simulink model "EcoSIM3_P2_C2_WIP"  (R2014b)
settings: Solver=ode1  SolverMode=SingleTasking  StartTime=0.0  StopTime=4  FixedStep=0.01  RelTol=1e-3
PostLoadFcn:
  | %, if any(exist('dsrtsu_mdlpostloadfcn', 'file') == [2, 3, 6]), try dsrtsu_mdlpostloadfcn('Execute', bdroot); catch fprintf('Error in PostLoadFcn (dsrtsu_mdlpostloadfcn) for model "%s":\n %s\n', bdroot, lasterr); end, end,
InitFcn:
  | tic
  | %Startup_EcoSIM
undefined symbols (not defined in the file or in its folder): canChannel, Controls, DriveCycles, Driver, EM_EFF_MAP, EM_PwrLoss_MAP, EngPwr, EngSpd, EngTrq, Glbl, Overwritten_Mode, Plants, Power, sigbuilder_block, Torque, Trialmap, Veh_Dynamics
libraries: simulink x135, canmsglib x113, fl_lib x104, canlib x89, nesl_utility x56, sdl_lib x29, dspsigops x6, dspswit3 x5, dspstat3 x2, commnoisgen2 x1, dspfdesign x1
(part 6 of 21)

== system EcoSIM3_P2_C2_WIP/Powertrain/Clutch_Transmission1/Mastershift Softecu/Algorithm ==
  note: Cignals getting transmitted to Actuators are bussed together here
  note: Sensor signals getting transmitted over CAN are selected here
  note: Signals like T& E are used to calculate whatever is required by Soft ECU
  Inputs : Inport
  Add4 : Sum
  Bus Creator : BusCreator  Inputs=2
  Bus Selector : BusSelector  OutputSignals=Clutch_Sw,Sensor_Out.Trans_Sensor_Out.Actual_Gear,Upshift_Sw,Downshift_Sw
  Chart : Stateflow chart  TreatAsAtomicUnit=on
  Display : Display
  Display1 : Display
  Downshift Counter : dspswit3/Counter  Direction=Up  CountEvent=Rising edge  CounterSize=User defined  MaxCount=255  InitialCount=0  Output=Count  HitValue=32  ResetInput=on  SamplesPerFrame=1  Ts=1  CntDtype=double  HitDtype=Logical
  Gain : Gain  Gain=-1
  Memory : Memory
  Memory1 : Memory
  Upshift Counter : dspswit3/Counter  Direction=Up  CountEvent=Rising edge  CounterSize=User defined  MaxCount=255  InitialCount=0  Output=Count  HitValue=32  ResetInput=on  SamplesPerFrame=1  Ts=1  CntDtype=double  HitDtype=Logical
  Outputs : Outport
  wires:
  Chart/1(Gear_Cmd) -> Bus Creator/1, Display/1
  Memory1/1 -> Upshift Counter/2, Downshift Counter/2
  Bus Creator/1 -> Outputs/1
  Memory/1 -> Chart/2(Actual_Gear)
  Chart/3(reset) -> Memory1/1  "reset"
  Add4/1 -> Display1/1, Chart/3(Count)
  Bus Selector/4 -> Downshift Counter/1  "<Downshift_Sw>"
  Bus Selector/3 -> Upshift Counter/1  "<Upshift_Sw>"
  Gain/1 -> Add4/2
  Downshift Counter/1 -> Gain/1
  Upshift Counter/1 -> Add4/1
  Chart/2(TCM_Gear) -> Bus Creator/2  "TCM_Gear"
  Bus Selector/1 -> Chart/1(Clutch_Sw)  "<Clutch_Sw>"
  Bus Selector/2 -> Memory/1  "<Actual_Gear>"
  Inputs/1 -> Bus Selector/1

== system EcoSIM3_P2_C2_WIP/Powertrain/Clutch_Transmission1/Mastershift Softecu/Inputs ==
  note: Combine all the Signals that go to the
      | Soft ECU Algorithm:
      | -Calculated Signals from Sensors and CAN
      | -Signalfrom sensors pass through because they
      | need to be sent out over the CAN by the ECU
  note: Select the Sensor signals
  note: Select the CAN signals
  note: Do the input conditioning (if any) required by the
      | Algorith
  Sensors : Inport
  From GCM : Inport  Port=2
  Clutch_CAN_Out : Inport  Port=3
  Bus Creator : BusCreator
  Bus Selector : BusSelector  OutputSignals=Upshift_Sw,Downshift_Sw
  Bus Selector1 : BusSelector  OutputSignals=Clutch_Sw
  To_Algorithm : Outport
  wires:
  Bus Selector/2 -> Bus Creator/3  "<Downshift_Sw>"
  Bus Selector/1 -> Bus Creator/2  "<Upshift_Sw>"
  Bus Selector1/1 -> Bus Creator/4  "<Clutch_Sw>"
  Clutch_CAN_Out/1 -> Bus Selector1/1
  Bus Creator/1 -> To_Algorithm/1  "Component_to_Alg"
  Sensors/1 -> Bus Creator/1
  From GCM/1 -> Bus Selector/1

== system EcoSIM3_P2_C2_WIP/Powertrain/Clutch_Transmission1/Mastershift Softecu/Outputs ==
  note: Combine all the Signals that go to the
      | Soft ECU Algorithm:
      | -Calculated Signals from Sensors and CAN
      | -Signalfrom sensors pass through because they
      | need to be sent out over the CAN by the ECU
  From Algorithm : Inport
  Bus Creator : BusCreator  Inputs=1
  Bus Selector : BusSelector  OutputSignals=Gear_Cmd,TCM_Gear
  Actuator Commands : Outport
  To GCM : Outport  Port=2
  wires:
  Bus Creator/1 -> Actuator Commands/1  "Trans_Actuator_Commands"
  Bus Selector/2 -> To GCM/1  "<TCM_Gear>"
  Bus Selector/1 -> Bus Creator/1  "<Gear_Cmd>"
  From Algorithm/1 -> Bus Selector/1

== system EcoSIM3_P2_C2_WIP/Powertrain/Clutch_Transmission1/Trans_Plant/Actuators ==
  note: Actuator Model or a Signal Pass-through, Remove the bus if you are passing through all the signals
  ActuatorInputs : Inport
  Actuator Outputs : Outport
  wires:
  ActuatorInputs/1 -> Actuator Outputs/1

== system EcoSIM3_P2_C2_WIP/Powertrain/Clutch_Transmission1/Trans_Plant/Plant ==
  note: Component Level Performance Maps
  note: Try to detect actual gears from simscape model. Using reverse lookup from rate limiter starts giving value from Gear 5, because it has the lowest ratio
  From_Actuators : Inport
  Bus Selector : BusSelector  OutputSignals=Clutch_Trans_SoftECU_Receive.Clutch_Trans_CAN.Trans_Receive.Gear_Request
  Input Shaft Inertia : fl_lib/Mechanical/Rotational Elements/Inertia  inertia=0.01 kg*m^2  w_specify=off  w_priority=High  w=580*2*pi/60 rad/s  t_specify=off  t_priority=High  t=0 N*m
  Output Shaft Inertia1 : fl_lib/Mechanical/Rotational Elements/Inertia  inertia=.01 kg*m^2  w_specify=off  w_priority=High  w=580*2*pi/60 rad/s  t_specify=off  t_priority=High  t=0 N*m
  Rate Limiter : RateLimiter  RisingSlewLimit=2  FallingSlewLimit=-2  SampleTimeMode=inherited  InitialCondition=2.95
  ReverseLookup : Lookup  InputValues=[0 0.6300 1 1.3400 1.9400 2.9500]  Table=[0 5 4 3 2 1]  LookUpMeth=Use Input Nearest
  Simulink-PS Converter : nesl_utility/Simulink-PS Converter  PhysicalDomain=network_engine_domain  SubClassName=ps_input  LeftPortType=input  RightPortType=output  PseudoPeriodic=off  Frequencies=[]  NoiseDistribution=none  NoiseParameters=[]  Unit=1  AffineConversion=off  InputFiltering=off  SimscapeFilterOrder=1  InputFilterTimeConstant=0.001  UdotUserProvided=1
  Trans GR : Lookup  InputValues=Plants.Trans.Mdl.Plant.Gear_cmd  Table=Plants.Trans.Mdl.Plant.GR  LookUpMeth=Use Input Nearest
  Variable Ratio Transmission : sdl_lib/Couplings & Drives/Variable Ratio Transmission  rotation_direction=1  kp=3e+5 N*m/rad  kv=0.05 N*m/(rad/s)  initial_torque=0 N*m  losses_model=1  efficiency=0.8  mu_visc=[ 0 0 ] N*m/(rad/s)  w_thr=0.01 rad/s
  Trans Input Shaft : PMIOPort  Port=1  Side=Left
  To Sensors : PMIOPort  Port=2  Side=Right
  Actual_Gear : Outport
  wires:
  Rate Limiter/1 -> Simulink-PS Converter/1, ReverseLookup/1
  Trans GR/1 -> Rate Limiter/1
  ReverseLookup/1 -> Actual_Gear/1
  From_Actuators/1 -> Bus Selector/1
  Bus Selector/1 -> Trans GR/1  "<Gear_Request>"
  connections:
  Simulink-PS Converter/RConn1 -- Variable Ratio Transmission/LConn1
  To Sensors/RConn1 -- Output Shaft Inertia1/LConn1 -- Variable Ratio Transmission/RConn1
  Variable Ratio Transmission/LConn2 -- Input Shaft Inertia/LConn1 -- Trans Input Shaft/RConn1

== system EcoSIM3_P2_C2_WIP/Powertrain/Clutch_Transmission1/Trans_Plant/Sensors ==
  note: Sensor Model: Place where we add Corrupter
  Actual_Gear : Inport
  Bus Creator : BusCreator  Inputs=3
  Ideal Rotational Motion Sensor : fl_lib/Mechanical/Mechanical Sensors/Ideal Rotational Motion Sensor  offset=0 rad
  Ideal Torque Sensor : fl_lib/Mechanical/Mechanical Sensors/Ideal Torque Sensor
  Mechanical Rotational Reference1 : fl_lib/Mechanical/Rotational Elements/Mechanical Rotational Reference
  PS-Simulink Converter : nesl_utility/PS-Simulink Converter  PhysicalDomain=network_engine_domain  SubClassName=ps_output  LeftPortType=input  RightPortType=output  PseudoPeriodic=off  Frequencies=[]  Unit=1  AffineConversion=off
  PS-Simulink Converter1 : nesl_utility/PS-Simulink Converter  PhysicalDomain=network_engine_domain  SubClassName=ps_output  LeftPortType=input  RightPortType=output  PseudoPeriodic=off  Frequencies=[]  Unit=N*m  AffineConversion=off
  Trans Output Shaft : PMIOPort  Port=1  Side=Left
  To_MC : PMIOPort  Tag=PMCPort  Port=2  Side=Right
  Sensor Out : Outport
  ActGear : Outport  Port=2
  wires:
  Actual_Gear/1 -> Bus Creator/1, ActGear/1  "Actual_Gear"
  PS-Simulink Converter/1 -> Bus Creator/2  "Trans_Speed_rad_per_s"
  PS-Simulink Converter1/1 -> Bus Creator/3  "Trans_Torque_Out_Nm"
  Bus Creator/1 -> Sensor Out/1  "Trans_Sensor"
  connections:
  Ideal Torque Sensor/LConn1 -- Ideal Rotational Motion Sensor/LConn1 -- Trans Output Shaft/RConn1
  Ideal Rotational Motion Sensor/RConn1 -- Mechanical Rotational Reference1/LConn1
  PS-Simulink Converter1/LConn1 -- Ideal Torque Sensor/RConn2
  PS-Simulink Converter/LConn1 -- Ideal Rotational Motion Sensor/RConn2
  To_MC/RConn1 -- Ideal Torque Sensor/RConn1

== system EcoSIM3_P2_C2_WIP/Powertrain/Clutch_Transmission2/CP1 SoftEcu/Algorithm ==
  note: Cignals getting transmitted to Actuators are bussed together here
  note: Sensor signals getting transmitted over CAN are bussed together here
  note: Sensor signals getting transmitted over CAN are selected here
  note: Signals like T& E are used to calculate whatever is required by Soft ECU
  note: SpA position 0 to 6327
      | 0 = Fully Engaged
      | 6327 = Fully Disengaged
  Inputs : Inport
  Add : Sum  Inputs=-+
  Bus Creator2 : BusCreator
  Bus Selector : BusSelector  OutputSignals=CP1_SoftECU_Receive.CP1_CAN.MSG_HYB_15.MY15_CCU_posDes,Sensor_Out.Clutch_Sensor_Out.Clutch_Pressure
  Chart : Stateflow chart  TreatAsAtomicUnit=on
  Constant : Constant
  Gain : Gain  Gain=1/6327
  Gain1 : Gain  Gain=1/(4400000*0.4)
  Gain2 : Gain  Gain=6327
  Ground : Ground
  Scope : Scope
      settings: SaveName=ScopeData51
  Scope1 : Scope
      settings: SaveName=ScopeData52
  Outputs : Outport
  wires:
  Inputs/1 -> Bus Selector/1
  Bus Selector/1 -> Scope1/1, Chart/1(Position_Request)  "<MY15_CCU_posDes>"
  Chart/2(Mode) -> Bus Creator2/2  "CY01_stMode"
  Chart/1(Position_Command) -> Gain/1
  Gain/1 -> Bus Creator2/1  "SpA_Position_Command"
  Gain1/1 -> Add/1
  Bus Selector/2 -> Gain1/1  "<Clutch_Pressure>"
  Gain2/1 -> Scope/1, Bus Creator2/3  "CY01_posCurr"
  Ground/1 -> Bus Creator2/4  "Dummy_Electrical1"
  Bus Creator2/1 -> Outputs/1  "CP1_SoftECU_Out"
  Add/1 -> Gain2/1
  Constant/1 -> Add/2

== system EcoSIM3_P2_C2_WIP/Powertrain/Clutch_Transmission2/CP1 SoftEcu/Inputs ==
  note: Combine all the Signals that go to the
      | Soft ECU Algorithm:
      | -Calculated Signals from Sensors and CAN
      | -Signalfrom sensors pass through because they
      | need to be sent out over the CAN by the ECU
  note: Select the Sensor signals
  note: Select the CAN signals
  note: Do the input conditioning (if any) required by the
      | Algorith
  Sensors : Inport
  CAN : Inport  Port=2
  Bus Creator : BusCreator  Inputs=2
  Bus Selector : BusSelector  OutputSignals=CP1_SoftECU_Receive
  To_Algorithm : Outport
  wires:
  Bus Creator/1 -> To_Algorithm/1  "Component_to_Alg"
  Sensors/1 -> Bus Creator/1  "Sensor_Out"
  CAN/1 -> Bus Selector/1
  Bus Selector/1 -> Bus Creator/2  "<CP1_SoftECU_Receive>"

== system EcoSIM3_P2_C2_WIP/Powertrain/Clutch_Transmission2/CP1 SoftEcu/Outputs ==
  From Algorithm : Inport
  Bus Creator : BusCreator  Inputs=1
  Bus Creator1 : BusCreator  Inputs=3
  Bus Selector1 : BusSelector  OutputSignals=SpA_Position_Command,CY01_stMode,CY01_posCurr,Dummy_Electrical1
  Actuator Cmd : Outport
  CAN : Outport  Port=2
  wires:
  From Algorithm/1 -> Bus Selector1/1  "Sensor_Out"
  Bus Selector1/1 -> Bus Creator/1  "<SpA_Position_Command>"
  Bus Creator/1 -> Actuator Cmd/1  "Component_Actuator_Commands"
  Bus Selector1/3 -> Bus Creator1/2  "<CY01_posCurr>"
  Bus Selector1/4 -> Bus Creator1/3  "<Dummy_Electrical1>"
  Bus Selector1/2 -> Bus Creator1/1  "<CY01_stMode>"
  Bus Creator1/1 -> CAN/1  "CP1_Out"

== system EcoSIM3_P2_C2_WIP/Powertrain/Clutch_Transmission2/Clutch_Plant/Custom Clutch ==
  -1 : fl_lib/Physical Signals/Functions/PS Gain  gain=-1
  Dynamic friction coefficient lookup table : fl_lib/Physical Signals/Lookup Tables/PS Lookup Table (1D)  x_t=[ 0 0.1 0.2 0.3 0.4 0.5 1 2 5 10 100 1000 ]  y_t=[ 0.29 0.28 0.26 0.22 0.21 0.2 0.2 0.19 0.19 0.19 0.19 0.19 ]  interp_method=1  extrap_method=1
  Effective radius : fl_lib/Physical Signals/Functions/PS Gain  gain=0.3
  Fundamental Friction Clutch : sdl_lib/Clutches/Fundamental Components/Fundamental Friction Clutch  unidirectional=0  w_tol=0.001 rad/s  initial_state_locked=0
  PS Abs : fl_lib/Physical Signals/Nonlinear Operators/PS Abs
  PS Product1 : fl_lib/Physical Signals/Functions/PS Product
  PS-Simulink Converter1 : nesl_utility/PS-Simulink Converter  PhysicalDomain=network_engine_domain  SubClassName=ps_output  LeftPortType=input  RightPortType=output  PseudoPeriodic=off  Frequencies=[]  Unit=rad/s  AffineConversion=off
  Peak force : fl_lib/Physical Signals/Functions/PS Gain  gain=10
  Slip(rad/s) : Scope
      settings: YMin=-4  YMax=1
  Static/dynamic friction ratio : fl_lib/Physical Signals/Functions/PS Gain  gain=1.1
  "[0, inf]" : fl_lib/Physical Signals/Nonlinear Operators/PS Saturation  upper_limit=inf  lower_limit=0
  P : PMIOPort  Port=1  Side=Left
  Mode : PMIOPort  Port=2  Side=Right
  F : PMIOPort  Port=3  Side=Right
  B : PMIOPort  Port=4  Side=Left
  wires:
  PS-Simulink Converter1/1 -> Slip(rad/s)/1
  connections:
  Peak force/RConn1 -- PS Product1/LConn1
  PS Product1/RConn1 -- Effective radius/LConn1
  "[0, inf]"/RConn1 -- Peak force/LConn1
  Fundamental Friction Clutch/RConn3 -- F/RConn1
  Fundamental Friction Clutch/RConn2 -- Mode/RConn1
  PS-Simulink Converter1/LConn1 -- Fundamental Friction Clutch/RConn1 -- PS Abs/LConn1
  B/RConn1 -- Fundamental Friction Clutch/LConn4
  P/RConn1 -- "[0, inf]"/LConn1
  Fundamental Friction Clutch/LConn2 -- -1/LConn1 -- Static/dynamic friction ratio/RConn1
  Effective radius/RConn1 -- Fundamental Friction Clutch/LConn1 -- Static/dynamic friction ratio/LConn1
  Dynamic friction coefficient lookup table/RConn1 -- PS Product1/LConn2
  -1/RConn1 -- Fundamental Friction Clutch/LConn3
  PS Abs/RConn1 -- Dynamic friction coefficient lookup table/LConn1

== system EcoSIM3_P2_C2_WIP/Powertrain/Clutch_Transmission2/Clutch_Plant/Sensors ==
  Clutch_Pressure : Inport
  Bus Creator : BusCreator  Inputs=1
  Ideal Rotational Motion Sensor : fl_lib/Mechanical/Mechanical Sensors/Ideal Rotational Motion Sensor  offset=0 rad
  Ideal Torque Sensor : fl_lib/Mechanical/Mechanical Sensors/Ideal Torque Sensor
  Mechanical Rotational Reference1 : fl_lib/Mechanical/Rotational Elements/Mechanical Rotational Reference
  PS-Simulink Converter : nesl_utility/PS-Simulink Converter  PhysicalDomain=network_engine_domain  SubClassName=ps_output  LeftPortType=input  RightPortType=output  PseudoPeriodic=off  Frequencies=[]  Unit=rad/s  AffineConversion=off
  PS-Simulink Converter1 : nesl_utility/PS-Simulink Converter  PhysicalDomain=network_engine_domain  SubClassName=ps_output  LeftPortType=input  RightPortType=output  PseudoPeriodic=off  Frequencies=[]  Unit=N*m  AffineConversion=off
  Terminator : Terminator
  Terminator1 : Terminator
  Shaft : PMIOPort  Port=1  Side=Left
  To_Trans : PMIOPort  Tag=PMCPort  Port=2  Side=Right
  Clutch_Status : Outport
  wires:
  PS-Simulink Converter/1 -> Terminator/1  "Clutch_Speed_rad_per_s"
  PS-Simulink Converter1/1 -> Terminator1/1  "Clutch_Torque_Out_Nm"
  Clutch_Pressure/1 -> Bus Creator/1  "Clutch_Pressure"
  Bus Creator/1 -> Clutch_Status/1  "Clutch_Sensor_Out"
  connections:
  Ideal Torque Sensor/LConn1 -- Shaft/RConn1 -- Ideal Rotational Motion Sensor/LConn1
  Ideal Rotational Motion Sensor/RConn1 -- Mechanical Rotational Reference1/LConn1
  PS-Simulink Converter/LConn1 -- Ideal Rotational Motion Sensor/RConn2
  PS-Simulink Converter1/LConn1 -- Ideal Torque Sensor/RConn2
  To_Trans/RConn1 -- Ideal Torque Sensor/RConn1

== system EcoSIM3_P2_C2_WIP/Powertrain/Clutch_Transmission2/Mastershift Softecu/Algorithm ==
  note: Signals like T& E are used to calculate whatever is required by Soft ECU
  note: Sensor signals getting transmitted over CAN are selected here
  note: Cignals getting transmitted to Actuators are bussed together here
  Inputs : Inport
  Add4 : Sum
  Bus Creator : BusCreator  Inputs=3
  Bus Selector : BusSelector  OutputSignals=Mastershift_SoftECU_Receive.Mastershift_Electrical.Clutch_Sw,Sensor_Out.Trans_Sensor_Out.Actual_Gear,Mastershift_SoftECU_Receive.Mastershift_Electrical.Upshift_Sw,Mastershift_SoftECU_Receive.Mastershift_Electrical.Downshift_Sw
  Chart : Stateflow chart  TreatAsAtomicUnit=on
  Display : Display
  Display1 : Display
  Downshift Counter : dspswit3/Counter  Direction=Up  CountEvent=Rising edge  CounterSize=User defined  MaxCount=255  InitialCount=0  Output=Count  HitValue=32  ResetInput=on  SamplesPerFrame=1  Ts=1  CntDtype=double  HitDtype=Logical
  Gain : Gain  Gain=-1
  Ground : Ground
  Memory : Memory
  Memory1 : Memory
  Scope : Scope
      settings: SaveName=ScopeData30
  Scope1 : Scope
      settings: SaveName=ScopeData31
  Scope2 : Scope
      settings: SaveName=ScopeData48
  Upshift Counter : dspswit3/Counter  Direction=Up  CountEvent=Rising edge  CounterSize=User defined  MaxCount=255  InitialCount=0  Output=Count  HitValue=32  ResetInput=on  SamplesPerFrame=1  Ts=1  CntDtype=double  HitDtype=Logical
  Outputs : Outport
  wires:
  Inputs/1 -> Bus Selector/1
  Bus Selector/2 -> Memory/1  "<Actual_Gear>"
  Bus Selector/1 -> Chart/1(Clutch_Sw)  "<Clutch_Sw>"
  Chart/2(TCM_Gear) -> Bus Creator/2  "Mastershift_Gear"
  Upshift Counter/1 -> Add4/1
  Downshift Counter/1 -> Gain/1
  Gain/1 -> Add4/2
  Bus Selector/3 -> Scope/1, Upshift Counter/1  "<Upshift_Sw>"
  Bus Selector/4 -> Downshift Counter/1  "<Downshift_Sw>"
  Add4/1 -> Scope1/1, Chart/3(Count), Display1/1
  Chart/3(reset) -> Memory1/1  "reset"
  Memory/1 -> Chart/2(Actual_Gear)
  Bus Creator/1 -> Outputs/1  "Mastershift_SoftECU_Out"
  Memory1/1 -> Downshift Counter/2, Upshift Counter/2
  Chart/1(Gear_Cmd) -> Scope2/1, Bus Creator/1, Display/1
  Ground/1 -> Bus Creator/3  "Dummy_Electrical1"

== system EcoSIM3_P2_C2_WIP/Powertrain/Clutch_Transmission2/Mastershift Softecu/Inputs ==
  note: Do the input conditioning (if any) required by the
      | Algorith
  note: Select the CAN signals
  note: Select the Sensor signals
  note: Combine all the Signals that go to the
      | Soft ECU Algorithm:
      | -Calculated Signals from Sensors and CAN
      | -Signalfrom sensors pass through because they
      | need to be sent out over the CAN by the ECU
  Sensors : Inport
  CAN : Inport  Port=2
  Bus Creator : BusCreator  Inputs=2
  Bus Selector : BusSelector  OutputSignals=Mastershift_SoftECU_Receive
  To_Algorithm : Outport
  wires:
  CAN/1 -> Bus Selector/1
  Sensors/1 -> Bus Creator/1
  Bus Creator/1 -> To_Algorithm/1  "Component_to_Alg"
  Bus Selector/1 -> Bus Creator/2  "<Mastershift_SoftECU_Receive>"

== system EcoSIM3_P2_C2_WIP/Powertrain/Clutch_Transmission2/Mastershift Softecu/Outputs ==
  note: Combine all the Signals that go to the
      | Soft ECU Algorithm:
      | -Calculated Signals from Sensors and CAN
      | -Signalfrom sensors pass through because they
      | need to be sent out over the CAN by the ECU
  From Algorithm : Inport
  Bus Creator : BusCreator  Inputs=1
  Bus Creator1 : BusCreator  Inputs=2
  Bus Selector : BusSelector  OutputSignals=Gear_Cmd,Mastershift_Gear,Dummy_Electrical1
  Actuator Commands : Outport
  CANTx : Outport  Port=2
  wires:
  From Algorithm/1 -> Bus Selector/1
  Bus Selector/1 -> Bus Creator/1  "<Gear_Cmd>"
  Bus Creator/1 -> Actuator Commands/1  "Trans_Actuator_Commands"
  Bus Selector/2 -> Bus Creator1/1  "<Mastershift_Gear>"
  Bus Selector/3 -> Bus Creator1/2  "<Dummy_Electrical1>"
  Bus Creator1/1 -> CANTx/1  "Mastershift_Out"

== system EcoSIM3_P2_C2_WIP/Powertrain/Clutch_Transmission2/Trans_Plant/Actuators ==
  note: Actuator Model or a Signal Pass-through, Remove the bus if you are passing through all the signals
  ActuatorInputs : Inport
  Actuator Outputs : Outport
  wires:
  ActuatorInputs/1 -> Actuator Outputs/1

== system EcoSIM3_P2_C2_WIP/Powertrain/Clutch_Transmission2/Trans_Plant/Plant ==
  note: Try to detect actual gears from simscape model. Using reverse lookup from rate limiter starts giving value from Gear 5, because it has the lowest ratio
  note: Component Level Performance Maps
  From_Actuators : Inport
  Bus Creator : BusCreator  Inputs=3
  Bus Selector : BusSelector  OutputSignals=Gear_Cmd
  Bus Selector1 : BusSelector  OutputSignals=Shaft_1-2_Dog_Clutch_posn_mm
  Bus Selector2 : BusSelector  OutputSignals=Shaft_5-R_Dog_Clutch_posn_mm
  Bus Selector3 : BusSelector  OutputSignals=Shaft_3-4_Dog_Clutch_posn_mm
  Display : Display
  Display1 : Display
  Display2 : Display
  Gear1-2 : Subsystem
  Gear3-4 : Subsystem
  Gear5-R : Subsystem
  Input Shaft Inertia : fl_lib/Mechanical/Rotational Elements/Inertia  inertia=0.01 kg*m^2  w_specify=off  w_priority=High  w=580*2*pi/60 rad/s  t_specify=off  t_priority=High  t=0 N*m
  Mux : Mux  Inputs=3
  Mux1 : Mux  Inputs=3
  Mux2 : Mux  Inputs=2
  Output Shaft Inertia1 : fl_lib/Mechanical/Rotational Elements/Inertia  inertia=.01 kg*m^2  w_specify=off  w_priority=High  w=580*2*pi/60 rad/s  t_specify=off  t_priority=High  t=0 N*m
  Rate Limiter1 : RateLimiter  Commented=on  RisingSlewLimit=2  FallingSlewLimit=-2  SampleTimeMode=inherited  InitialCondition=2.95
  ReverseLookup : Lookup  Commented=on  InputValues=[0 0.6300 1 1.3400 1.9400 2.9500]  Table=[0 5 4 3 2 1]  LookUpMeth=Use Input Nearest
  Rounding Function : Rounding
  Scope : Scope  Commented=on
      settings: SaveName=ScopeData28
  Scope{1..5} (5 alike) : Scope
      Scope1 settings: SaveName=ScopeData29
      Scope2 settings: SaveName=ScopeData2
      Scope4 settings: SaveName=ScopeData4
  Simulink-PS Converter : nesl_utility/Simulink-PS Converter  Commented=on  PhysicalDomain=network_engine_domain  SubClassName=ps_input  LeftPortType=input  RightPortType=output  PseudoPeriodic=off  Frequencies=[]  NoiseDistribution=none  NoiseParameters=[]  Unit=1  AffineConversion=off  InputFiltering=off  SimscapeFilterOrder=1  InputFilterTimeConstant=0.001  UdotUserProvided=1
  Subsystem : Subsystem
  Trans GR : Lookup  Commented=on  InputValues=Plants.Trans.Mdl.Plant.Gear_cmd  Table=Plants.Trans.Mdl.Plant.GR  LookUpMeth=Use Input Nearest
  Transport Delay : TransportDelay  Commented=on  DelayTime=0.1
  Truth Table : Truth Table  TreatAsAtomicUnit=on
  Variable Ratio Transmission : sdl_lib/Couplings & Drives/Variable Ratio Transmission  Commented=on  rotation_direction=1  kp=3e+5 N*m/rad  kv=0.05 N*m/(rad/s)  initial_torque=0 N*m  losses_model=1  efficiency=0.8  mu_visc=[ 0 0 ] N*m/(rad/s)  w_thr=0.01 rad/s
  Trans Input Shaft : PMIOPort  Port=1  Side=Left
  To Sensors : PMIOPort  Port=2  Side=Right
  Actual_Gear : Outport
  wires:
  From_Actuators/1 -> Bus Selector/1
  Trans GR/1 -> Rate Limiter1/1
  Rate Limiter1/1 -> ReverseLookup/1, Simulink-PS Converter/1
  Mux2/1 -> Scope2/1
  Bus Selector2/1 -> Display2/1, Mux/1  "<Shaft_5-R_Dog_Clutch_posn_mm>"
  Mux/1 -> Scope5/1
  Bus Selector3/1 -> Mux/3, Display/1  "<Shaft_3-4_Dog_Clutch_posn_mm>"
  Gear3-4/1(ShaftPosn) -> Bus Creator/2, Bus Selector3/1
  Bus Selector1/1 -> Mux/2, Display1/1  "<Shaft_1-2_Dog_Clutch_posn_mm>"
  Gear1-2/1(ShaftPosn) -> Bus Creator/3, Bus Selector1/1
  Truth Table/3(y1) -> Mux1/3, Gear1-2/1(In1)
  Truth Table/1(y3) -> Mux1/1, Gear5-R/1(In1)
  Rounding Function/1 -> Scope3/1, Mux2/1, Truth Table/1(u)
  Subsystem/1(Out1) -> Actual_Gear/1, Mux2/2  "Actual_Gear"
  Bus Creator/1 -> Subsystem/1(In1)
  Truth Table/2(y2) -> Mux1/2, Gear3-4/1(In1)
  Mux1/1 -> Scope4/1
  Gear5-R/1(ShaftPosn) -> Bus Creator/1, Bus Selector2/1
  Bus Selector/1 -> Rounding Function/1  "<Gear_Cmd>"
  connections:
  Gear5-R/LConn1 -- Gear1-2/LConn1 -- Trans Input Shaft/RConn1 -- Input Shaft Inertia/LConn1 -- Gear3-4/LConn1
  Gear5-R/RConn1 -- To Sensors/RConn1 -- Output Shaft Inertia1/LConn1 -- Gear1-2/RConn1 -- Gear3-4/RConn1

== system EcoSIM3_P2_C2_WIP/Powertrain/Clutch_Transmission2/Trans_Plant/Sensors ==
  note: Sensor Model: Place where we add Corrupter
  Actual_Gear : Inport
  Bus Creator : BusCreator  Inputs=3
  Ideal Rotational Motion Sensor : fl_lib/Mechanical/Mechanical Sensors/Ideal Rotational Motion Sensor  offset=0 rad
  Ideal Torque Sensor : fl_lib/Mechanical/Mechanical Sensors/Ideal Torque Sensor
  Mechanical Rotational Reference1 : fl_lib/Mechanical/Rotational Elements/Mechanical Rotational Reference
  PS-Simulink Converter : nesl_utility/PS-Simulink Converter  PhysicalDomain=network_engine_domain  SubClassName=ps_output  LeftPortType=input  RightPortType=output  PseudoPeriodic=off  Frequencies=[]  Unit=1  AffineConversion=off
  PS-Simulink Converter1 : nesl_utility/PS-Simulink Converter  PhysicalDomain=network_engine_domain  SubClassName=ps_output  LeftPortType=input  RightPortType=output  PseudoPeriodic=off  Frequencies=[]  Unit=N*m  AffineConversion=off
  Trans Output Shaft : PMIOPort  Port=1  Side=Left
  To_MC : PMIOPort  Tag=PMCPort  Port=2  Side=Right
  Sensor Out : Outport
  wires:
  Bus Creator/1 -> Sensor Out/1  "Trans_Sensor"
  PS-Simulink Converter1/1 -> Bus Creator/3  "Trans_Torque_Out_Nm"
  PS-Simulink Converter/1 -> Bus Creator/2  "Trans_Speed_rad_per_s"
  Actual_Gear/1 -> Bus Creator/1  "Actual_Gear"
  connections:
  To_MC/RConn1 -- Ideal Torque Sensor/RConn1
  PS-Simulink Converter/LConn1 -- Ideal Rotational Motion Sensor/RConn2
  PS-Simulink Converter1/LConn1 -- Ideal Torque Sensor/RConn2
  Mechanical Rotational Reference1/LConn1 -- Ideal Rotational Motion Sensor/RConn1
  Trans Output Shaft/RConn1 -- Ideal Rotational Motion Sensor/LConn1 -- Ideal Torque Sensor/LConn1

== system EcoSIM3_P2_C2_WIP/Powertrain/Electric Motor / Component Model/Actuators ==
  note: Actuator Model or a Signal Pass-through, Remove the bus if you are passing through all the signals
  ActuatorInputs : Inport
  Bus Creator : BusCreator  Inputs=1
  Bus Selector : BusSelector  OutputSignals=Commanded_Torque
  Gain : Gain
  Actuator Outputs : Outport
  wires:
  ActuatorInputs/1 -> Bus Selector/1
  Bus Selector/1 -> Gain/1  "<Commanded_Torque>"
  Gain/1 -> Bus Creator/1  "EM_Torque_Request_Nm"
  Bus Creator/1 -> Actuator Outputs/1

== system EcoSIM3_P2_C2_WIP/Powertrain/Electric Motor / Component Model/Plant ==
  note: Earlier 0.2
  note: Checked the setting 'Use Fixed-cost run time' after adding Double synchro blocks. Otherwise non convergence would terminate the simulation.
  note: Component Level Performance Maps
  note: Three kinds of Outputs:
      | 1.To_sensors: Signals that can actually be sensed through Sensors go to sensor models
      | 2. To_plants: Signals that are not actually sensed by sensors but are utilized by the rest of the plant and actually happen physically
      | Component_Logging: Logs both the signal kinds before going through sensor
  note: Component Level Performance Maps
  From_Actuators : Inport
  Sensor_Feedback : Inport  Port=2
  Bias : Bias  Bias=-1
  Bus Creator : BusCreator  Inputs=2
  Bus Selector : BusSelector  OutputSignals=EM_Torque_Request_Nm
  Bus Selector1 : BusSelector  OutputSignals=EM_Speed_produced_rad_per_s
  Bus Selector2 : BusSelector  OutputSignals=Simulation_mode
  Constant : Constant  Value=130/277.3
  Constant1 : Constant
  EM Efficiency : Lookup2D  Commented=on  RowIndex=Plants.EM.Mdl.Plant.w_rad  ColumnIndex=Plants.EM.Mdl.Plant.T_Nm  Table=Plants.EM.Mdl.Plant.Eff  LookUpMeth=Interpolation-Use End Values  SaturateOnIntegerOverflow=on  InputSameDT=on
  EM Max Torque Curve : Lookup  InputValues=Plants.EM.Mdl.Plant.max_min_w  Table=Plants.EM.Mdl.Plant.T_max_Peak  LookUpMeth=Interpolation-Use End Values  SaturateOnIntegerOverflow=on
  EM Min Torque Curve : Lookup  InputValues=Plants.EM.Mdl.Plant.max_min_w  Table=Plants.EM.Mdl.Plant.T_min_Peak  LookUpMeth=Interpolation-Use End Values  SaturateOnIntegerOverflow=on
  EM Power Loss : Lookup2D  RowIndex=Plants.EM.Mdl.Plant.w_rad_PL  ColumnIndex=Plants.EM.Mdl.Plant.T_Nm_PL  Table=Plants.EM.Mdl.Plant.power_loss  LookUpMeth=Interpolation-Use End Values  SaturateOnIntegerOverflow=on  InputSameDT=on
  EM_Thermal_Model : Subsystem
  Gain : Gain  Gain=0.93
  Ideal Torque Source1 : fl_lib/Mechanical/Mechanical Sources/Ideal Torque Source
  Inertia1 : fl_lib/Mechanical/Rotational Elements/Inertia  inertia=0.02825 kg*m^2  w_specify=off  w_priority=High  w=0 rad/s  t_specify=off  t_priority=High  t=0 N*m
  InternalMotorError : Constant  Value=0
  Mechanical Rotational Reference1 : fl_lib/Mechanical/Rotational Elements/Mechanical Rotational Reference
  Product : Product
  Saturation Dynamic1 : simulink/Discontinuities/Saturation Dynamic  OutMin=[]  OutMax=[]  OutDataTypeStr=Inherit: Same as second input  OutDataType=sfix(16)  OutScaling=2^-10  DoSatur=off
  Scope : Scope
      settings: SaveName=ScopeData60
  Simulink-PS Converter1 : nesl_utility/Simulink-PS Converter  PhysicalDomain=network_engine_domain  SubClassName=ps_input  LeftPortType=input  RightPortType=output  PseudoPeriodic=off  Frequencies=[]  NoiseDistribution=none  NoiseParameters=[]  Unit=N*m  AffineConversion=off  InputFiltering=off  SimscapeFilterOrder=1  InputFilterTimeConstant=.001  UdotUserProvided=1
  Solver Configuration1 : nesl_utility/Solver Configuration  PhysicalDomain=network_engine_domain  SubClassName=solver  LeftPortType=input  RightPortType=generic  Accelerate=off  Tones=[]  Harmonics=[]  SimulateNoise=off  Profile=off  UseLocalSampling=off  EnableSwitchedLinearOptims=on  FrequencyDomain=off  UseCCode=off  RelTol=0.001  AbsTol=1e-06  MinStep=1e-09  ToWorkspace=off  DoDC=off  ResidualTolerance=1e-9  UseLocalSolver=on  LocalSolverChoice=NE_BACKWARD_EULER_ADVANCER  LocalSolverSampleTime=0.01  DoFixedCost=on  MaxNonlinIter=3  MaxModeIter=2  LinearAlgebra=Sparse  DelaysMemoryBudget=1024  AutomaticFiltering=on  FilteringTimeConstant=0.001
  Switch : Switch  Criteria=u2 > Threshold  Threshold=0.5
  To_Plants1 : PMIOPort  Port=1  Side=Right
  To_Sensors : Outport
  wires:
  Bus Creator/1 -> To_Sensors/1  "EM_to_sensors"
  From_Actuators/1 -> Bus Selector/1
  Product/1 -> Saturation Dynamic1/1
  EM Min Torque Curve/1 -> Saturation Dynamic1/3
  Bus Selector/1 -> Saturation Dynamic1/2  "<EM_Torque_Request_Nm>"
  InternalMotorError/1 -> Bus Creator/1  "InternalMotorError"
  Sensor_Feedback/1 -> Bus Selector1/1
  Bus Selector1/1 -> EM Max Torque Curve/1, EM Min Torque Curve/1, EM Power Loss/1  "<EM_Speed_produced_rad_per_s>"
  Saturation Dynamic1/1 -> EM Power Loss/2, Scope/1, Simulink-PS Converter1/1
  EM Power Loss/1 -> EM_Thermal_Model/1(EM_Power_Loss)  "EM_Power_Loss"
  EM_Thermal_Model/1(Out1) -> Bus Creator/2
  EM Max Torque Curve/1 -> Gain/1
  [Simulation_Parameters] -> Bus Selector2/1
  Bus Selector2/1 -> Bias/1  "<Simulation_mode>"
  Bias/1 -> Switch/2
  Constant/1 -> Switch/1
  Constant1/1 -> Product/1, Switch/3
  Gain/1 -> Product/2
  connections:
  Simulink-PS Converter1/RConn1 -- Ideal Torque Source1/RConn1
  Ideal Torque Source1/LConn1 -- To_Plants1/RConn1 -- Inertia1/LConn1 -- Solver Configuration1/RConn1
  Ideal Torque Source1/RConn2 -- Mechanical Rotational Reference1/LConn1

== system EcoSIM3_P2_C2_WIP/Powertrain/Electric Motor / Component Model/Sensors ==
  note: Sensor Model: Place where we add Corrupter
  Sensor In : Inport
  Bus Creator : BusCreator  Inputs=5
  Bus Selector : BusSelector  OutputSignals=InternalMotorError,EM_Temperature_degC
  Bus Selector1 : BusSelector  OutputSignals=EM_Torque_Produced_Nm,EM_Speed_produced_rad_per_s
  Fault Insertation : Subsystem
  Ideal Rotational Motion Sensor : fl_lib/Mechanical/Mechanical Sensors/Ideal Rotational Motion Sensor  offset=0 rad
  Ideal Torque Sensor : fl_lib/Mechanical/Mechanical Sensors/Ideal Torque Sensor
  Mechanical Rotational Reference1 : fl_lib/Mechanical/Rotational Elements/Mechanical Rotational Reference
  PS-Simulink Converter : nesl_utility/PS-Simulink Converter  PhysicalDomain=network_engine_domain  SubClassName=ps_output  LeftPortType=input  RightPortType=output  PseudoPeriodic=off  Frequencies=[]  Unit=1  AffineConversion=off
  PS-Simulink Converter1 : nesl_utility/PS-Simulink Converter  PhysicalDomain=network_engine_domain  SubClassName=ps_output  LeftPortType=input  RightPortType=output  PseudoPeriodic=off  Frequencies=[]  Unit=1  AffineConversion=off
  Product : Product
  Scope : Scope
      settings: SaveName=ScopeData59
  Sensor lag : Subsystem
  Sensor lag1 : Subsystem
  Sensors : Subsystem
  Terminator : Terminator
  Shaft : PMIOPort  Port=1  Side=Left
  To_Plants : PMIOPort  Port=2  Side=Right
  Sensor Out : Outport
  To_Battery : Outport  Port=2
  wires:
  Bus Creator/1 -> Sensor Out/1  "EM_Sensor_Out"
  Sensor In/1 -> Bus Selector/1
  Bus Selector/1 -> Bus Creator/1  "<InternalMotorError>"
  Sensor lag/1(o) -> Terminator/1  "EM_Speed_rad_per_s"
  Sensor lag1/1(o) -> Scope/1, Fault Insertation/1(In1), Bus Creator/4  "EM_Torque_Out_Nm"
  Product/1 -> Bus Creator/5, To_Battery/1  "EM_Power_In_W"
  PS-Simulink Converter1/1 -> Sensor lag1/1(i)  "EM_Torque_Out_Nm"
  PS-Simulink Converter/1 -> Sensor lag/1(i)  "EM_Speed_rad_per_s"
  Sensors/1(EM_Shaft_out) -> Bus Selector1/1
  Bus Selector1/1 -> Product/1  "<EM_Torque_Produced_Nm>"
  Bus Selector1/2 -> Product/2, Bus Creator/3  "<EM_Speed_produced_rad_per_s>"
  Bus Selector/2 -> Bus Creator/2  "<EM_Temperature_degC>"
  connections:
  Shaft/RConn1 -- Ideal Rotational Motion Sensor/LConn1 -- Ideal Torque Sensor/LConn1
  Ideal Rotational Motion Sensor/RConn1 -- Mechanical Rotational Reference1/LConn1
  PS-Simulink Converter/LConn1 -- Ideal Rotational Motion Sensor/RConn2
  PS-Simulink Converter1/LConn1 -- Ideal Torque Sensor/RConn2
  Sensors/LConn1 -- Fault Insertation/RConn1 -- Ideal Torque Sensor/RConn1
  To_Plants/RConn1 -- Sensors/RConn1

== system EcoSIM3_P2_C2_WIP/Powertrain/Electric Motor /Soft ECU/Algorithm ==
  note: The batt_mainc_stat used by this model is actually the
      | bcm_mainc_stat signal transmitted by the ESS softECU
  note: Sensor signals getting transmitted over CAN are selected here
  note: Feedback signals from the Normal state. Signals contain RUN_Fault and ShutdownRequest
  Inputs : Inport
  Bus Creator1 : BusCreator  Inputs=2
  Compare To Constant : simulink/Logic and Bit Operations/Compare To Constant  relop===  const=6  OutDataTypeStr=boolean
  Inputs1 : InportShadow
  Normal Operation : Subsystem
  Rinehart Documentation : Subsystem
      settings: OpenFcn=open('/Component_docs/RMS CAN Protocol (V4_0).pdf')
  Startup_Shutdown : Subsystem
  Outputs : Outport
  wires:
  Bus Creator1/1 -> Outputs/1  "EM_Out"
  Normal Operation/1(Status) -> Bus Creator1/2, Startup_Shutdown/2(Faults)
  Compare To Constant/1 -> Normal Operation/Enable
  Inputs/1 -> Startup_Shutdown/1(SignalIn)
  [EM_Torque_Cmd_Trigger] -> Normal Operation/2(FaultTrigger)
  Startup_Shutdown/2(VSM) -> Compare To Constant/1
  Startup_Shutdown/1(Inverter_Status) -> Bus Creator1/1
  Inputs1/1 -> Normal Operation/1(SignalIn)

== system EcoSIM3_P2_C2_WIP/Powertrain/Electric Motor /Soft ECU/Inputs ==
  note: Change Name according to protocol, thats what the .dbc names should be
  note: Do the input conditioning (if any) required by the
      | Algorith
  note: Select the CAN signals
  note: Select the Sensor signals
  note: Combine all the Signals that go to the
      | Soft ECU Algorithm:
      | -Calculated Signals from Sensors and CAN
      | -Signalfrom sensors pass through because they
      | need to be sent out over the CAN by the ECU
  From_ECUs : Inport
  Sensors : Inport  Port=2
  Bus Creator : BusCreator  Inputs=3
  Bus Creator1 : BusCreator
  Bus Selector : BusSelector  OutputSignals=EM_CAN_Messages,ESS_Transmit.ESS_CAN_Out
  Bus Selector1 : BusSelector  OutputSignals=EM_Temperature_degC,InternalMotorError,EM_Speed_produced_rad_per_s,EM_Torque_Out_Nm
  Gain : Gain
  To_Algorithm : Outport
  wires:
  From_ECUs/1 -> Bus Selector/1
  Sensors/1 -> Bus Selector1/1
  Bus Creator/1 -> To_Algorithm/1  "Component_to_Alg"
  Bus Selector/1 -> Bus Creator/2  "<EM_CAN_Messages>"
  Bus Selector1/3 -> Gain/1  "<EM_Speed_produced_rad_per_s>"
  Gain/1 -> Bus Creator1/3  "Motor_Speed"
  Bus Creator1/1 -> Bus Creator/1  "EM_Sensors"
  Bus Selector1/2 -> Bus Creator1/2  "<InternalMotorError>"
  Bus Selector/2 -> Bus Creator/3  "<ESS_CAN_Out>"
  Bus Selector1/4 -> Bus Creator1/4  "<EM_Torque_Out_Nm>"
  Bus Selector1/1 -> Bus Creator1/1  "<EM_Temperature_degC>"

== system EcoSIM3_P2_C2_WIP/Powertrain/Electric Motor /Soft ECU/Outputs ==
  note: Change Name according to protocol, thats what the .dbc names should be
  From Algorithm : Inport
  Bus Creator1 : BusCreator  Inputs=1
  Bus Selector : BusSelector  OutputSignals=RunningStatus.Commanded_Torque
  To_ECUs : Outport
  Actuator Commands : Outport  Port=2
  wires:
  Bus Creator1/1 -> Actuator Commands/1  "EM_Actuator_Cmds"
  From Algorithm/1 -> Bus Selector/1, To_ECUs/1
  Bus Selector/1 -> Bus Creator1/1  "<Commanded_Torque>"

== system EcoSIM3_P2_C2_WIP/Powertrain/Electrical Storage System/ ESS Model/Actuators ==
  note: The switch is emulating the battery contactor:
      | If the bcm_manc_stat is less than 1 there will be no power request from the ESS
  note: This is I*V Requested
  note: Actuator Model or a Signal Pass-through, Remove the bus if you are passing through all the signals
  ActuatorInputs : Inport
  Charger_P_in [W] : Inport  Port=2
  EM P_in [W] : Inport  Port=3
  Acc P_in [W] : Inport  Port=4
  BAS P_in [W] : Inport  Port=5
  Add : Sum  Inputs=++++
  Bus Creator : BusCreator  Inputs=2
  Bus Selector : BusSelector  OutputSignals=Contactors_Closed
  Contactors : Switch  Criteria=u2 > Threshold  Threshold=0.5
  ESS_Power_Request : Constant  Value=0
  Scope : Scope
      settings: SaveName=ScopeData3
  Actuator Outputs : Outport
  wires:
  ActuatorInputs/1 -> Bus Creator/1, Bus Selector/1
  EM P_in [W]/1 -> Add/2
  BAS P_in [W]/1 -> Add/4
  Contactors/1 -> Scope/1, Bus Creator/2  "Component_Power_Request_W"
  Bus Creator/1 -> Actuator Outputs/1  "Component_Power_Request_W"
  Bus Selector/1 -> Contactors/2  "<Contactors_Closed>"
  Add/1 -> Contactors/1  "Component_Power_Request_W"
  ESS_Power_Request/1 -> Contactors/3
  Charger_P_in [W]/1 -> Add/1
  Acc P_in [W]/1 -> Add/3

== system EcoSIM3_P2_C2_WIP/Powertrain/Electrical Storage System/ ESS Model/Plant ==
  note: Three kinds of Outputs:
      | 1.To_sensors: Signals that can actually be sensed through Sensors go to sensor models
      | 2. To_plants: Signals that are not actually sensed by sensors but are utilized by the rest of the plant and actually happen physically
      | Component_Logging: Logs both the signal kinds before going through sensor
  note: BATTERY MODEL
  From_Actuators : Inport
  Bus Creator : BusCreator  Inputs=5
  Bus Selector : BusSelector  OutputSignals=ESS_Actuator_Cmds.AccPwrMdlHiVltInpCrnt,Component_Power_Request_W
  Electrical Plant Model : Subsystem
  Integrator : Integrator
  Power Calculation : Subsystem
  Scope : Scope
      settings: SaveName=ScopeData74
  Terminator1 : Terminator
  Terminator2 : Terminator
  Thermal Model : Subsystem
  To_Sensors : Outport
  wires:
  Bus Creator/1 -> To_Sensors/1  "ESS_to_sensors"
  From_Actuators/1 -> Bus Selector/1
  Electrical Plant Model/1(Batt_Current [A]) -> Integrator/1, Bus Creator/2
  Electrical Plant Model/2(Batt_SOC [%]) -> Bus Creator/3
  Electrical Plant Model/3(Batt_volt [V]) -> Bus Creator/4
  Thermal Model/1(Batt_Temp [C]) -> Scope/1, Electrical Plant Model/2(Batt_Temp [C]), Bus Creator/5
  Bus Selector/1 -> Power Calculation/1(Input_Crnt [A])  "<AccPwrMdlHiVltInpCrnt>"
  Power Calculation/1(P_in [W]) -> Electrical Plant Model/1(P_in [W])
  Electrical Plant Model/5(Batt_volt_1 [V]) -> Power Calculation/2(Batt_volt_1 [V])
  Electrical Plant Model/4(Batt_Heat [W]) -> Thermal Model/1(Batt_Heat [W])
  Integrator/1 -> Bus Creator/1  "BATT_cap_used"
  Power Calculation/2(Batt_Electrical_Energy) -> Terminator1/1
  Power Calculation/3(Batt_Electrical_Energy_Net) -> Terminator2/1
  Bus Selector/2 -> Power Calculation/3(Component_Power_Watts)  "<Component_Power_Request_W>"

== system EcoSIM3_P2_C2_WIP/Powertrain/Electrical Storage System/ ESS Model/Sensors ==
  note: Sensor Model: Place where we add Corrupter
  Sensor In : Inport
  Bus Creator : BusCreator
  Bus Selector : BusSelector  OutputSignals=Batt_Current_A,Batt_SOC_percent,Batt_Temp_C,Batt_Voltage_V
  Sensor Out : Outport
  wires:
  Bus Creator/1 -> Sensor Out/1  "ESS_Sensor_Out"
  Sensor In/1 -> Bus Selector/1
  Bus Selector/1 -> Bus Creator/1  "<Batt_Current_A>"
  Bus Selector/2 -> Bus Creator/2  "<Batt_SOC_percent>"
  Bus Selector/3 -> Bus Creator/3  "<Batt_Temp_C>"
  Bus Selector/4 -> Bus Creator/4  "<Batt_Voltage_V>"

== system EcoSIM3_P2_C2_WIP/Powertrain/Electrical Storage System/Soft ECU/Algorithm ==
  note: Signals like T& E are used to calculate whatever is required by Soft ECU
  note: bcm_cell_tmax coming from sensors = temperature of hottest cell in the pack
  note: Discharge buffer only based on temperature
  Inputs : Inport
  A123 BMS : Stateflow chart  TreatAsAtomicUnit=on
  A123 Documentation : Subsystem
      settings: OpenFcn=open('/Component_docs/EcoCAR A123 ICD v1.pdf')
  Bus Creator : BusCreator  Inputs=18
  Bus Selector : BusSelector  OutputSignals=AccPwrMdlHiVltInpCrnt,Component_Sensor_Out.Batt_SOC_percent,Component_Sensor_Out.Batt_Voltage_V,Component_Sensor_Out.Batt_Current_A,BMS_Powerup,hsc_bcm_enable,hsc_bcm_mainc_close,Component_Sensor_Out.Batt_Temp_C,hsc_bcm_epo,hsc_bcm_leakage_ena,veh_wake,chga_wake,Component_Sensor_Out.Batt_Temp_C
  Compare To Constant : simulink/Logic and Bit Operations/Compare To Constant  relop=>=  const=95  OutDataTypeStr=boolean
  Constant : Constant  Value=60
  Constant1 : Constant  Value=-40
  Current Buffer : Subsystem
  Data Type Conversion : DataTypeConversion
  Data Type Conversion1 : DataTypeConversion
  Discharge buffer : Lookup_n-D  NumberOfTableDimensions=1  BreakpointsForDimension1=[-40 10 45 48 58 60]  Table=[0 100 100 90 20 0]  ExtrapMethod=Clip  UseLastTableValue=on  InternalRulePriority=Speed  RndMeth=Simplest  InputSameDT=on
  Gain : Gain
  Gain1 : Gain  Gain=0.8
  Scope : Scope
      settings: SaveName=ScopeData65
  Scope1 : Scope
      settings: SaveName=ScopeData66
  Subsystem : Subsystem
  Terminator : Terminator
  Terminator1 : Terminator
  Outputs : Outport
  wires:
  Gain1/1 -> Bus Creator/7  "bcm_cell_tmin"
  Bus Selector/4 -> Current Buffer/1(Current), Bus Creator/5  "<Batt_Current_A>"
  Bus Selector/3 -> Bus Creator/4  "<Batt_Voltage_V>"
  Data Type Conversion1/1 -> Bus Creator/3  "bcm_chg_done"
  Bus Selector/2 -> Compare To Constant/1, Bus Creator/2  "<Batt_SOC_percent>"
  Bus Selector/1 -> Bus Creator/1  "<AccPwrMdlHiVltInpCrnt>"
  Subsystem/10(Out10) -> Bus Creator/17
  Subsystem/9(Out9) -> Bus Creator/16
  Subsystem/8(Out8) -> Bus Creator/15
  Subsystem/7(Out7) -> Bus Creator/14
  Subsystem/6(Out6) -> Bus Creator/13
  Subsystem/5(Out5) -> Bus Creator/12
  Subsystem/4(Out4) -> Bus Creator/11
  Subsystem/3(Out3) -> Bus Creator/10
  Subsystem/2(Out2) -> Bus Creator/9
  Subsystem/1(Out1) -> Bus Creator/8
  A123 BMS/10(bcm_on_plug) -> Subsystem/10(In10)
  A123 BMS/9(chga_ena) -> Subsystem/9(In9)
  A123 BMS/8(bcm_veh_mon) -> Subsystem/8(In8)
  A123 BMS/7(bcm_epo) -> Subsystem/7(In7)  "bcm_epo"
  A123 BMS/6(bcm_cpwr_mon) -> Subsystem/6(In6)  "bcm_cpwr_mon"
  A123 BMS/5(bcm_cpwr_cmd) -> Subsystem/5(In5)  "bcm_cpwr_cmd"
  A123 BMS/4(bcm_chgc_stat) -> Subsystem/4(In4)  "bcm_chgc_stat"
  A123 BMS/3(bcm_mainc_stat) -> Subsystem/3(In3)  "bcm_mainc_stat"
  A123 BMS/2(bcm_hvil_mon) -> Subsystem/2(In2)  "bcm_hvil_mon"
  A123 BMS/1(bcm_ready) -> Subsystem/1(In1)  "bcm_ready"
  Discharge buffer/1 -> Bus Creator/18, A123 BMS/9(bcm_dis_buffer)  "bcm_dis_buf"
  Gain/1 -> Gain1/1, Bus Creator/6, A123 BMS/4(bcm_cell_temp)  "bcm_cell_tmax"
  Bus Selector/13 -> Discharge buffer/1  "<Batt_Temp_C>"
  Data Type Conversion/1 -> A123 BMS/12(Charger_On)
  [Charger_On] -> Data Type Conversion/1
  Bus Selector/8 -> Gain/1  "<Batt_Temp_C>"
  Bus Selector/5 -> A123 BMS/1(PowerUp)  "<BMS_Powerup>"
  Bus Selector/10 -> A123 BMS/6(hsc_bcm_leakage_ena)  "<hsc_bcm_leakage_ena>"
  Bus Creator/1 -> Outputs/1  "ESS_SoftECU_Out"
  Bus Selector/9 -> A123 BMS/5(hsc_bcm_epo)  "<hsc_bcm_epo>"
  Constant1/1 -> A123 BMS/11(bcm_cell_t_lower_lim)
  Constant/1 -> A123 BMS/10(bcm_cell_t_upper_lim)
  Bus Selector/7 -> A123 BMS/3(hsc_bcm_mainc_close)  "<hsc_bcm_mainc_close>"
  Bus Selector/6 -> A123 BMS/2(hsc_bcm_enable)  "<hsc_bcm_enable>"
  Inputs/1 -> Bus Selector/1
  Bus Selector/11 -> A123 BMS/7(veh_wake)  "<veh_wake>"
  Bus Selector/12 -> A123 BMS/8(chga_wake)  "<chga_wake>"
  Compare To Constant/1 -> Data Type Conversion1/1  "bcm_chg_done"
  Current Buffer/1(charge buffer) -> Scope/1, Terminator/1
  Current Buffer/2(discharge buffer) -> Scope1/1, Terminator1/1

== system EcoSIM3_P2_C2_WIP/Powertrain/Electrical Storage System/Soft ECU/Inputs ==
  note: Do the input conditioning (if any) required by the
      | Algorith
  note: Select the CAN signals
  note: Select the Sensor signals
  note: Combine all the Signals that go to the
      | Soft ECU Algorithm:
      | -Calculated Signals from Sensors and CAN
      | -Signalfrom sensors pass through because they
      | need to be sent out over the CAN by the ECU
  Sensors : Inport
  CAN_In : Inport  Port=2
  Bus Creator : BusCreator  Inputs=9
  Bus Selector : BusSelector  OutputSignals=AccPwrMdlHiVltInpCrnt,hsc_bcm_mainc_close,hsc_bcm_enable,hsc_bcm_leakage_ena,hsc_bcm_epo,BMS_Powerup,chga_wake,veh_wake
  To_Algorithm : Outport
  wires:
  CAN_In/1 -> Bus Selector/1
  Sensors/1 -> Bus Creator/1
  Bus Creator/1 -> To_Algorithm/1  "Component_to_Alg"
  Bus Selector/1 -> Bus Creator/2  "<AccPwrMdlHiVltInpCrnt>"
  Bus Selector/2 -> Bus Creator/3  "<hsc_bcm_mainc_close>"
  Bus Selector/3 -> Bus Creator/4  "<hsc_bcm_enable>"
  Bus Selector/4 -> Bus Creator/5  "<hsc_bcm_leakage_ena>"
  Bus Selector/5 -> Bus Creator/6  "<hsc_bcm_epo>"
  Bus Selector/6 -> Bus Creator/7  "<BMS_Powerup>"
  Bus Selector/7 -> Bus Creator/8  "<chga_wake>"
  Bus Selector/8 -> Bus Creator/9  "<veh_wake>"

== system EcoSIM3_P2_C2_WIP/Powertrain/Electrical Storage System/Soft ECU/Outputs ==
  note: Select the Sensor signals
  From Algorithm : Inport
  Bus Creator3 : BusCreator  Inputs=2
  Bus Selector : BusSelector  OutputSignals=AccPwrMdlHiVltInpCrnt,bcm_mainc_stat,bcm_chgc_stat
  Data Type Conversion : DataTypeConversion
  Logical Operator : Logic  Operator=OR  IconShape=distinctive  AllPortsSameDT=off  OutDataTypeStr=boolean
  Actuator_Cmds : Outport
  To ECUs : Outport  Port=2
  wires:
  Bus Selector/1 -> Bus Creator3/1  "<AccPwrMdlHiVltInpCrnt>"
  From Algorithm/1 -> To ECUs/1, Bus Selector/1
  Bus Creator3/1 -> Actuator_Cmds/1  "ESS_Actuator_Cmds"
  Bus Selector/3 -> Logical Operator/2  "<bcm_chgc_stat>"
  Bus Selector/2 -> Logical Operator/1  "<bcm_mainc_stat>"
  Logical Operator/1 -> Data Type Conversion/1
  Data Type Conversion/1 -> Bus Creator3/2  "Contactors_Closed"

== system EcoSIM3_P2_C2_WIP/Powertrain/Engine/ Component Model/Actuators ==
  note: Actuator Model or a Signal Pass-through, Remove the bus if you are passing through all the signals
  ActuatorInputs : Inport
  Actuator Outputs : Outport
  wires:
  ActuatorInputs/1 -> Actuator Outputs/1
